simulink model "blockDiagramTask3"  (R2025a)
settings: Solver=VariableStepAuto  StartTime=0.0  StopTime=0.001  RelTol=1e-3
InitFcn:
  | run motor_specs.m
model workspace: external: MATLAB File motor_specs.m (data not in the file)
values from neighbouring files (symbols this model uses):
  A = [(-R/L), (-K_E/L); K_M/J, (-b/J)]    [motor_specs.m]    (also in ssAndTF.m = -((K_M*K_E + (C_V*R))/(J*R)))
  b = C_V / rpm_to_rs    (= 1.05042262441e-05)    [motor_specs.m]
  B = [(1/L), 0]'    [motor_specs.m]    (also in ssAndTF.m = [(1/L), 0; 0, (-1/J)])
  C = [0, 1]    [motor_specs.m]    (also in ssAndTF.m = [1, 0; 0, 1])
  D = 0    [motor_specs.m]    (also in ssAndTF.m = zeros(2,2))
  J = 6.3E-6    (= 6.3e-06)    [motor_specs.m]
  K_E = 0.006741/rpm_to_rs    (= 0.0643718082829)    [motor_specs.m]
  K_M = 0.0644    [motor_specs.m]
  L = 0.000238    [motor_specs.m]
  R = 3.23    [motor_specs.m]
  U_N = 36    [motor_specs.m]
libraries: fl_lib x3, ee_lib x2, nesl_utility x2, slpidlib x1
settings Model: Creator=josef  LastModifiedBy=josef

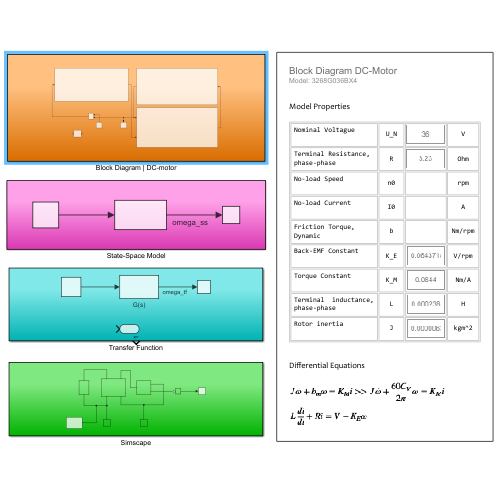
[thumbnail: Simulink's stored preview of the top-level diagram]
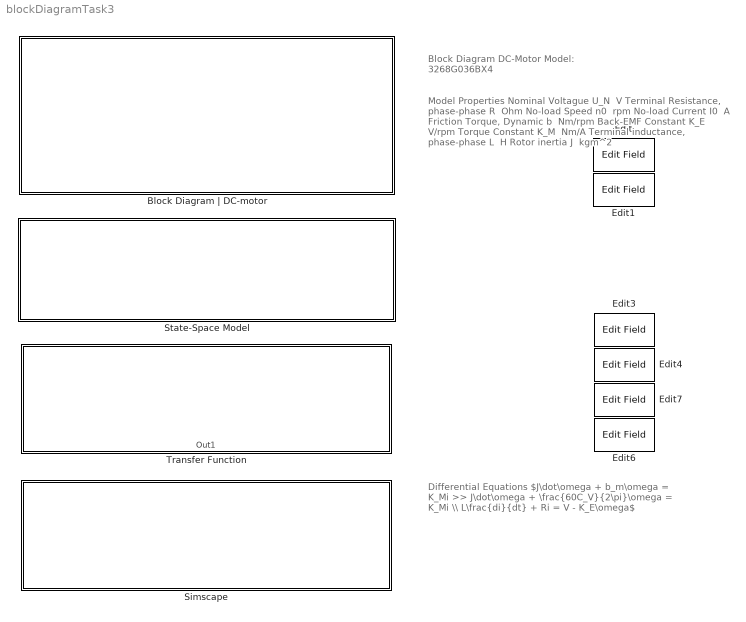
== system blockDiagramTask3 ==
  note: Differential Equations
      |
      | $J\dot\omega + b_m\omega = K_Mi >> J\dot\omega + \frac{60C_V}{2\pi}\omega = K_Mi \\ L\frac{di}{dt} + Ri = V - K_E\omega$
  note: Model Properties
      |
      | Nominal Voltague
      |
      | U_N
      | ​
      | V
      |
      | Terminal Resistance,
      | phase-phase
      | R
      | ​
      | Ohm
      |
      | No-load Speed
      |
      | n0
      | ​
      | rpm
      |
      | No-load Current
      |
      | I0
      | ​
      | A
      |
      | Friction Torque,
      | Dynamic
      | b
      | ​
      | Nm/rpm
      |
      | Back-EMF Constant
      |
      | K_E
      | ​
      | V/rpm
      |
      | Torque Constant
      |
      | K_M
      | ​
      | Nm/A
      |
      | Terminal inductance,
      | phase-phase
      | L
      | ​
      | H
      |
      | Rotor inertia
      |
      | J
      | ​
      | kgm^2
  note: Block Diagram DC-Motor
      | Model: 3268G036BX4
  Block Diagram | DC-motor : Subsystem
  Edit{,1,3..4,6..7} (6 alike) : EditField  LabelPosition=Hide  ShowInitialText=on  Alignment=Center  Opacity=0
  Simscape : Subsystem
  State-Space Model : Subsystem
  Transfer Function : Subsystem
      settings: PortSchema="{\"entries\":[{\"content\":{\"sides\":[{\"content\":{},\"type\":\"ConnectorPlacement.EquallySpacedRectSide\",\"uuid\":\"0067924e-7db0-4570-a079-fb467fb46ef4\"},{\"content\":{\"side\":\"RIGHT\"},\"type\":\"ConnectorPlacement.EquallySpacedRectSide\",\"uuid\":\"87851a09-b228-43ed-a4d6-92c4a38ec7d6\"},{\"content\":{\"side\":\"TOP\"},\"type\":\"ConnectorPlacement.EquallySpacedRectSide\",\"uuid\":\"37d2f610-147c-4c58-a6df-904738f34b04\"},{\"content\":{\"connectorIds\":[\"Out1\"],\"side\":\"BOTTOM\"},\"type\":\"ConnectorPlacement.EquallySpacedRectSide\",\"uuid\":\"d2131294-148d-4d1e-a5f3-2113a1d0f88b\"}]},\"type\":\"ConnectorPlacement.EquallySpacedConnector\",\"uuid\":\"c83b745b-613a-416d-9871-fba437cd355d\"}],\"packageUris\":[\"http://schema.mathworks.com/mf0/Connector/R2020b\"],\"version\":\"1.0\"}"

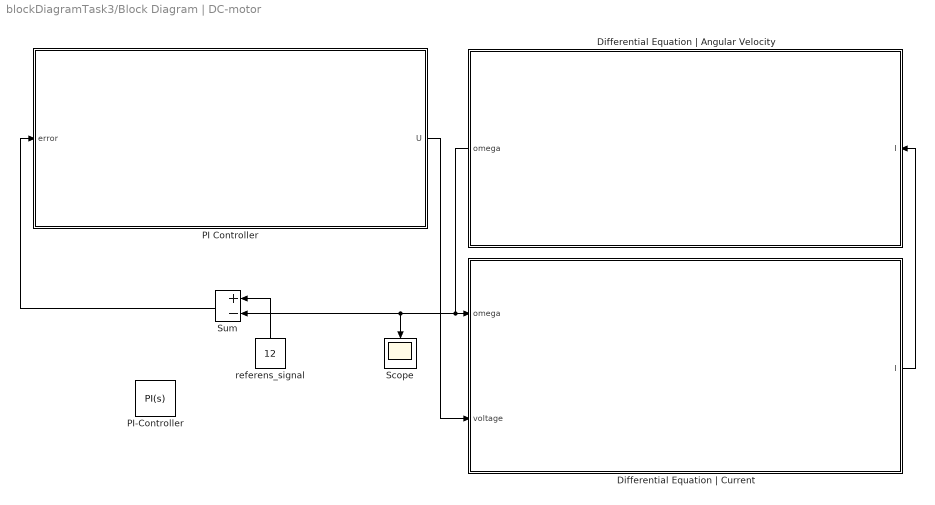
== system blockDiagramTask3/Block Diagram | DC-motor ==
  Differential Equation | Angular Velocity : Subsystem
  Differential Equation | Current : Subsystem
  PI Controller : Subsystem
  PI-Controller : slpidlib/PID Controller  Controller=PI  Form=Parallel  TimeDomain=Continuous-time  UseExternalTs=off  SampleTime=-1  IntegratorMethod=Forward Euler  FilterMethod=Forward Euler  ControllerParametersSource=internal  P=1.927  I=1  UseKiTs=off  D=0  UseExternalDerivativeSource=off  N=100  UseFilter=on  TunerSelectOption=Transfer Function Based (PID Tuner App)  InitialConditionSource=internal  InitialConditionForIntegrator=0  InitialConditionForFilter=0  DifferentiatorICPrevScaledInput=0  ExternalReset=none  TrackingMode=off  Kt=1  LimitOutput=off  SatLimitsSource=internal  UpperSaturationLimit=inf  LowerSaturationLimit=-inf  LinearizeAsGain=on  AntiWindupMode=none  Kb=1  LimitIntegrator=off  UpperIntegratorSaturationLimit=inf  LowerIntegratorSaturationLimit=-inf  POutMin=[]  POutMax=[]  IOutMin=[]  IOutMax=[]  DOutMin=[]  DOutMax=[]  NOutMin=[]  NOutMax=[]  SumOutMin=[]  SumOutMax=[]  SaturationOutMin=[]  SaturationOutMax=[]  PParamMin=[]  PParamMax=[]  IParamMin=[]  IParamMax=[]  DParamMin=[]  DParamMax=[]  NParamMin=[]  NParamMax=[]  KbParamMin=[]  KbParamMax=[]  KtParamMin=[]  KtParamMax=[]  KbOutMin=[]  KbOutMax=[]  KtOutMin=[]  KtOutMax=[]  IntegratorOutMin=[]  IntegratorOutMax=[]  FilterOutMin=[]  FilterOutMax=[]  SumI1OutMin=[]  SumI1OutMax=[]  SumI2OutMin=[]  SumI2OutMax=[]  SumI3OutMin=[]  SumI3OutMax=[]  SumI4OutMin=[]  SumI4OutMax=[]  SumDOutMin=[]  SumDOutMax=[]  DifferentiatorOutMin=[]  DifferentiatorOutMax=[]  FilterDiffOutCoefMin=[]  FilterDiffOutCoefMax=[]  ReciprocalOutMin=[]  ReciprocalOutMax=[]  SumDenOutMin=[]  SumDenOutMax=[]  SumNumOutMin=[]  SumNumOutMax=[]  DivideOutMin=[]  DivideOutMax=[]  UdiffTsProdOutMin=[]  UdiffTsProdOutMax=[]  NTsProdOutMin=[]  NTsProdOutMax=[]  UintegralTsProdOutMin=[]  UintegralTsProdOutMax=[]  UngainTsProdOutMin=[]  UngainTsProdOutMax=[]  ClampingZeroOutDataTypeStr=Inherit: Inherit via back propagation  ClampingZeroOutMin=[]  ClampingZeroOutMax=[]  FilterDenConstantOutDataTypeStr=Inherit: Inherit via back propagation  FilterDenConstantOutMin=[]  FilterDenConstantOutMax=[]  PCopyOutDataTypeStr=Inherit: Inherit via back propagation  PCopyOutMin=[]  PCopyOutMax=[]  NCopyOutDataTypeStr=Inherit: Inherit via back propagation  NCopyOutMin=[]  NCopyOutMax=[]  IntegratorContinuousStateAttributes=''  IntegratorStateMustResolveToSignalObject=off  IntegratorRTWStateStorageClass=Auto  FilterContinuousStateAttributes=''  FilterStateMustResolveToSignalObject=off  FilterRTWStateStorageClass=Auto  ParallelPVariant=InternalParameters  IdealPVariant=Disabled  IVariant=InternalParameters  DVariant=Disabled  IntegratorVariant=Continuous  SatVariant=Disabled  AWVariant=Passthrough  PCopyVariant=Disabled  TRVariant=Disabled  FdbkBlocksVariant=Forward  IdealPFdbkVariant=Disabled  SatFdbkVariant=Disabled  DerivativeFilterVariant=Disabled  NVariant=Disabled  NCopyVariant=Disabled_SignalSpec  FilterICVariant=Disabled  IntegratorICVariant=InternalICs  ExternalResetVariant=Disabled  TRSumVariant=Passthrough  SumFdbkVariant=Disabled  SumVariant=Sum_PI  TsampFilterVariant=InternalTs  TsampNgainVariant=Passthrough  TsampIntegralVariant=Disabled_SignalSpec  ExternalSaturationOutDataTypeStr=Inherit: Same as second input  DerivativeSourceVariant=Disabled  PreIntVariant=InternalPreInt
  Scope : Scope
      settings: ActiveDisplayYMinimum=-1.7692863504540333  ActiveDisplayYMaximum=15.923577154086303
  Sum : Sum  Inputs=+-
  referens_signal : Constant  Value=12
  wires:
  Differential Equation | Current/1(I) -> Differential Equation | Angular Velocity/1(I)
  referens_signal/1 -> Sum/1
  Differential Equation | Angular Velocity/1(omega) -> Sum/2, Scope/1, Differential Equation | Current/1(omega)
  Sum/1 -> PI Controller/1(error)
  PI Controller/1(U) -> Differential Equation | Current/2(voltage)

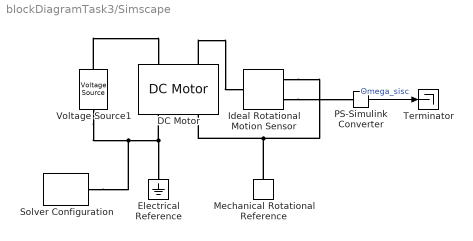
== system blockDiagramTask3/Simscape ==
  DC Motor : ee_lib/Electromechanical/Brushed Motors/DC Motor  field_option=ee.enum.field_option.pm  Rf=100 Ohm  Lf=1 H  Laf=0.15 H  If0=0 A  parameterization=ee.enum.dcparam_option.circuit_param  Ra=R Ohm  La=L H  emf_or_torque=ee.enum.emf_or_torque.kv  Kv=K_E V*s/rad  Ki=6.876e-4 N*m/A  T_stall=0.24e-3 N*m  w_max=19100 rpm  w_rated=15000 rpm  P_rated=0.08 W  V_rated=1.5 V  lam_param=ee.enum.lam_param.damping  i_noload=0 A  V_i_noload=1.5 V  J=J kg*m^2  lam=b N*m*s/rad  speed0=0 rpm  alpha=3.93e-3 1/K  Tmeas=25 degC  thermal_mass=100 J/K  initial_temperature=25 degC
  Electrical Reference : fl_lib/Electrical/Electrical Elements/Electrical Reference
  Ideal Rotational Motion Sensor : fl_lib/Mechanical/Mechanical Sensors/Ideal Rotational Motion Sensor  reference=foundation.enum.MeasurementReference.difference  acceleration_port=false  velocity_port=true  position_port=false  wrap_angle=false  offset=0 rad
      settings: InternalSimscapePortConfiguration="{\"Bottom\":[],\"Left\":[{\"id\":\"R\",\"label\":\"R\",\"type\":\"foundation.mechanical.rotational.rotational\"}],\"Right\":[{\"id\":\"C\",\"label\":\"C\",\"type\":\"foundation.mechanical.rotational.rotational\"},{\"id\":\"W\",\"label\":\"W\",\"type\":\"output\"}],\"Top\":[]}"
  Mechanical Rotational Reference : fl_lib/Mechanical/Rotational Elements/Mechanical Rotational Reference
  PS-Simulink Converter : nesl_utility/PS-Simulink Converter  PhysicalDomain=network_engine_domain  SubClassName=ps_output  LeftPortType=input  RightPortType=output  PseudoPeriodic=off  Frequencies=[]  VectorFormat=inherit  Unit=inherit  AffineConversion=off
  Solver Configuration : nesl_utility/Solver Configuration  PhysicalDomain=network_engine_domain  SubClassName=solver  LeftPortType=input  RightPortType=generic  Tones=[]  Harmonics=[]  SimulateNoise=off  Profile=off  UseLocalSampling=off  EnableSwitchedLinearOptims=on  FrequencyDomain=off  UseCCode=off  RelTol=0.001  AbsTol=0.001  MinStep=1e-09  ToWorkspace=off  RevertToSquareIcSolve=off  NumHomotopyIterations=100  PhasorMode=off  PhasorModeNumHarmonics=1  ConsistencySolver=NEWTON_XTOL_AFTER_FTOL  IndexReductionMethod=DerivativeReplacement  DoDC=off  ResidualTolerance=1e-09  ConsistencyTolSource=GLOBAL  ConsistencyAbsTol=0.001  ConsistencyRelTol=0.001  ConsistencyTolFactor=0.001  UseLocalSolver=off  LocalSolverChoice=NE_BACKWARD_EULER_ADVANCER  ResolveIndetEquations=on  FunctionEvalNumThread=1  LocalSolverSampleTime=0.001  DoFixedCost=off  MaxNonlinIter=3  MaxModeIter=2  ComputeImpulses=off  ImpulseIterations=2  LinearAlgebra=auto  LinearAlgebraNumThread=0  EquationFormulation=NE_TIME_EF  DelaysMemoryBudget=1024  AutomaticFiltering=on  FilteringTimeConstant=0.001  PartitionStorageMethod=AS_NEEDED  PartitionMemoryBudget=1024  PartitionMethod=ROBUST  MultibodyUseLocalSolver=off  MultibodyLocalSolverChoice=ODE1  MultibodyLocalSolverSampleTime=0.001
  Terminator : Terminator
  Voltage Source1 : ee_lib/Sources/Voltage Source  dc_voltage=U_N V  ac_voltage=0 V  ac_shift=0 rad  ac_frequency=60 Hz  noise_mode=ee.enum.sources.noise.Disabled  PSD=0 V^2/Hz  sample_time=1e-3 s  repeatability=ee.enum.sources.repeatability.NotRepeatable  user_seed=0  auto_seed=3890346746  i_specify=off  i_priority=None  i=0 A  i_nominal_specify=off  i_nominal_value=1  i_nominal_unit=A  v_specify=off  v_priority=None  v=0 V  v_nominal_specify=off  v_nominal_value=1  v_nominal_unit=V
  wires:
  PS-Simulink Converter/1 -> Terminator/1  "Omega_sisc"
  connections:
  Voltage Source1/RConn1 -- Solver Configuration/RConn1 -- Electrical Reference/LConn1 -- DC Motor/RConn1
  Ideal Rotational Motion Sensor/RConn1 -- Mechanical Rotational Reference/LConn1 -- DC Motor/RConn2
  DC Motor/LConn2 -- Ideal Rotational Motion Sensor/LConn1
  Voltage Source1/LConn1 -- DC Motor/LConn1
  Ideal Rotational Motion Sensor/RConn2 -- PS-Simulink Converter/LConn1

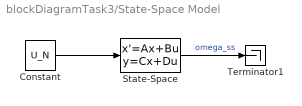
== system blockDiagramTask3/State-Space Model ==
  Constant : Constant  Value=U_N
  State-Space : StateSpace  A=A  B=B  C=C  D=D  InitialCondition=0
  Terminator1 : Terminator
  wires:
  State-Space/1 -> Terminator1/1  "omega_ss"
  Constant/1 -> State-Space/1

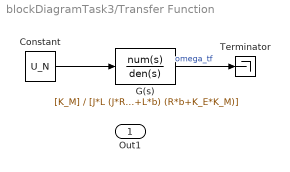
== system blockDiagramTask3/Transfer Function ==
  Constant : Constant  Value=U_N
  G(s) : TransferFcn  Numerator=[K_M]  Denominator=[J*L (J*R+L*b) (R*b+K_E*K_M)]
  Terminator : Terminator
  Out1 : Outport
  wires:
  G(s)/1 -> Terminator/1  "omega_tf"
  Constant/1 -> G(s)/1

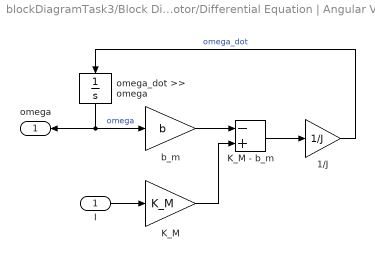
== system blockDiagramTask3/Block Diagram | DC-motor/Differential Equation | Angular Velocity ==
  I : Inport
  1/J : Gain  Gain=1/J
  K_M : Gain  Gain=K_M
  K_M - b_m : Sum  Inputs=-+
  b_m : Gain  Gain=b
  omega_dot >> omega : Integrator
  omega : Outport
  wires:
  b_m/1 -> K_M - b_m/1
  omega_dot >> omega/1 -> omega/1, b_m/1  "omega"
  K_M/1 -> K_M - b_m/2
  K_M - b_m/1 -> 1/J/1
  I/1 -> K_M/1
  1/J/1 -> omega_dot >> omega/1  "omega_dot"

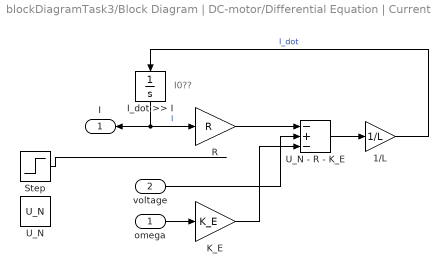
== system blockDiagramTask3/Block Diagram | DC-motor/Differential Equation | Current ==
  note: I0??
  omega : Inport
  voltage : Inport  Port=2
  1/L : Gain  Gain=1/L
  I_dot >> I : Integrator
  K_E : Gain  Gain=K_E
  R : Gain  Gain=R
  Step : Step  Time=0.0000001  After=36  SampleTime=0
  U_N : Constant  Value=U_N
  U_N - R - K_E : Sum  Inputs=-+-
  I : Outport
  wires:
  I_dot >> I/1 -> R/1, I/1  "I"
  K_E/1 -> U_N - R - K_E/3
  U_N - R - K_E/1 -> 1/L/1
  omega/1 -> K_E/1
  R/1 -> U_N - R - K_E/1
  1/L/1 -> I_dot >> I/1  "I_dot"
  Step/1 -> ?
  voltage/1 -> U_N - R - K_E/2

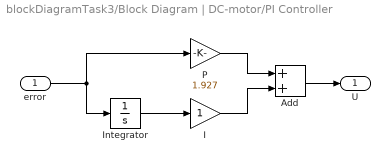
== system blockDiagramTask3/Block Diagram | DC-motor/PI Controller ==
  error : Inport
  Add : Sum
  I : Gain
  Integrator : Integrator
  P : Gain  Gain=1.927
  U : Outport
  wires:
  error/1 -> Integrator/1, P/1
  P/1 -> Add/1
  I/1 -> Add/2
  Add/1 -> U/1
  Integrator/1 -> I/1
